simulink model "AFSK"  (R2024b)
settings: Solver=VariableStepAuto  StartTime=0  StopTime=phi_LOS.Time(end)  RelTol=1e-3
PreLoadFcn:
  | addpath('./inputs')
  | 
  | fc = 120e3;
  | delta_f = 1000; % Hz
  | f0 = fc-(delta_f/2);
  | f1 = fc+(delta_f/2);
  | 
  | Rb = 1200; % bit rate = 1,2 kbps
  | Tb = 1/Rb; % Bit period = Frame period
  | Nc = 4; % the number of samples between 0 and 2π of the carrier. There are 100 periods in each Ns samples.
  | Ns = fc*Tb*Nc; % = 400 The number of samples per Tb.
  | Tsamp = Tb/Ns; % Sample period
  | Rsamp = 1/Tsamp; % sampling rate
  | 
  | fd = delta_f/2; % Frequency deviation
  | h = 2*fd*Tb; % Indice de modulação (h=5/6)
  | 
  | impulse_response = get_matched_filter_impulse_response(Tsamp, Tb, Ns, h);
  | [all_phases, odd_phases, even_phases] = get_phases(h);
  | % `terminal_phases` is `all_phases` reshaped to be used
  | % in the Viterbi algorithm during the metric computation
  | terminal_phases = repmat(cat(3, odd_phases.', even_phases.'), [1, 2, 1]);
  | N_terminal_phases = length(all_phases);
  | % Viterbi delay
  | K = 25;
  | 
  | % uplink frequency
  | f_uplink = 149e6;
  | 
  | % get real satellite orbits from `scintpy`
  | scenarios = get_scenarios();
  | %% Programmatically changable settings
  | % NOTE: don't put these variables in InitFcn. Otherwise,
  | % programmatic simulations will not work. If you want
  | % to change these varuables manually, use the command
  | % window, instead.
  | scenario = scenarios(1);
  | is_Doppler_realistic = true;
InitFcn:
  | % get realistic ϕ_LOS (in rad) and tau_LOS (in sec) (both sampled in Tb)
  | [phi_LOS, tau_LOS]= get_LOS_effects(f_uplink, scenario, Tb);
  | % get initial estimates
  | initial_estimates = get_initial_estimates(phi_LOS.Data, Tb);
  | % tau in number of symbols (unitless, sampled  in Tb)
  | tau_LOS_symbols = tau_LOS/Tb;
  | % 𝜏 LOS in in number of samples (unitless, sampled in Tb)
  | tau_LOS_samples = tau_LOS_symbols*Ns;
  | 
  | % you can change it in the manual switch
  | EbN0 = str2double(get_param('AFSK/AWGN Channel', 'EbNo'));
  | 
  | %% Kalman filter configurations
  | 
  | if is_Doppler_realistic
  |     x_00 = initial_estimates;
  | 
  |     % The transmmitted bit is delayed by `(init_LOS_delay+1)*Tb`
  |     % seconds to be it is compared with the detected bits,
  |     % where `init_LOS_delay` is the floor of the maximum LOS
  |     % delay that happens during the simulation. The delay
  |     % estimation operates to estimate the (likely) fractional
  |     % part between `(init_LOS_delay+1)*Tb` and the real LOS delay
  |     % that is occuring. This difference is fed back so that the
  |     % receive is (ideally) always delayed in `(init_LOS_delay+1)*Tb`
  |     % seconds as well. When it happens, the timing delay
  |     % estimation is working in lock.
  |     init_LOS_delay = floor(max(tau_LOS_symbols.Data));
  | 
  |     fprintf("The satellite name run in Simulnk model is %s\n", scenario.sat_name);
  | else
  |     nu_synthetic = str2double(get_param('AFSK/nu', 'Value'));
  |     nu_dot_synthetic = str2double(get_param('AFSK/nu_dot', 'Value'));
  |     x_00 = [0 nu_synthetic nu_dot_synthetic];
  |     init_LOS_delay = 0;
  | 
  |     fprintf("Simulnk model is running for dummy scenario with Doppler shift and drift given by %d Hz and %d Hz/s,respectively\n",...
  |         nu_synthetic, nu_dot_synthetic);
  | end
  | 
  | % Taylor Series truncation order
  | M = 3;
  | sigma2_process = [zeros(1,M-1),1e-2];
  | [Px_0_0,x00_matrix,Fk,Qk,Hk,Rk] = get_kf_intial_cfg(EbN0, M, Tb, sigma2_process, x_00, init_LOS_delay);
undefined symbols (not defined in the file): all_phases, dspblkCoreblockFVToolHelper, Fk, gcbh, Hk, phi, Px_0_0, Qk, real_tau_LOS, Rk, x00_matrix
libraries: dspswit3 x8, dspstat3 x4, simulink x4, dspsigops x2, commchan3 x1, commrandsrc3 x1, dspfdesign x1, dspinverses x1, commsink2 x1
settings Model: SimulationMode=rapid-accelerator  Creator=Rubem Pacelli  LastModifiedBy=felix
settings SolverCC: AlgebraicLoopSolver=TrustRegion
settings DataIOCC: SaveFormat=Structure  SaveOutput=off  SignalLogging=off  DSMLogging=off  SaveTime=off  ReturnWorkspaceOutputs=off
settings DebuggingCC: UnconnectedInputMsg=warning  UnconnectedOutputMsg=warning  UnconnectedLineMsg=warning  ArithmeticOperatorsInVariantConditions=warning
settings ModelReferenceCC: EnableRefExpFcnMdlSchedulingChecks=on
settings SFSimCC: SimUseLocalCustomCode=off  CustomCodeUndefinedFunction=UseInterfaceOnly
settings RTWCC: RTWUseLocalCustomCode=off  GPUComputeCapability=3.5  DLArmComputeVersion=19.05

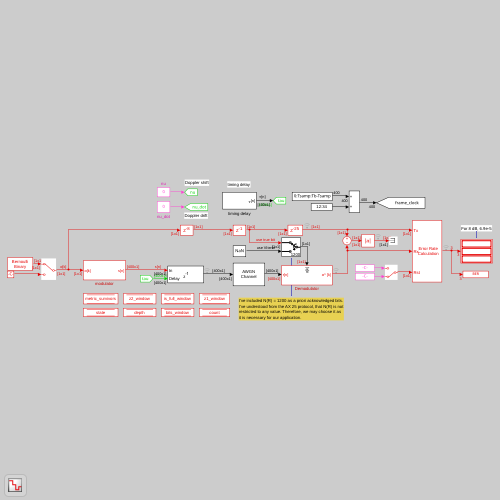
[thumbnail: Simulink's stored preview of the top-level diagram]
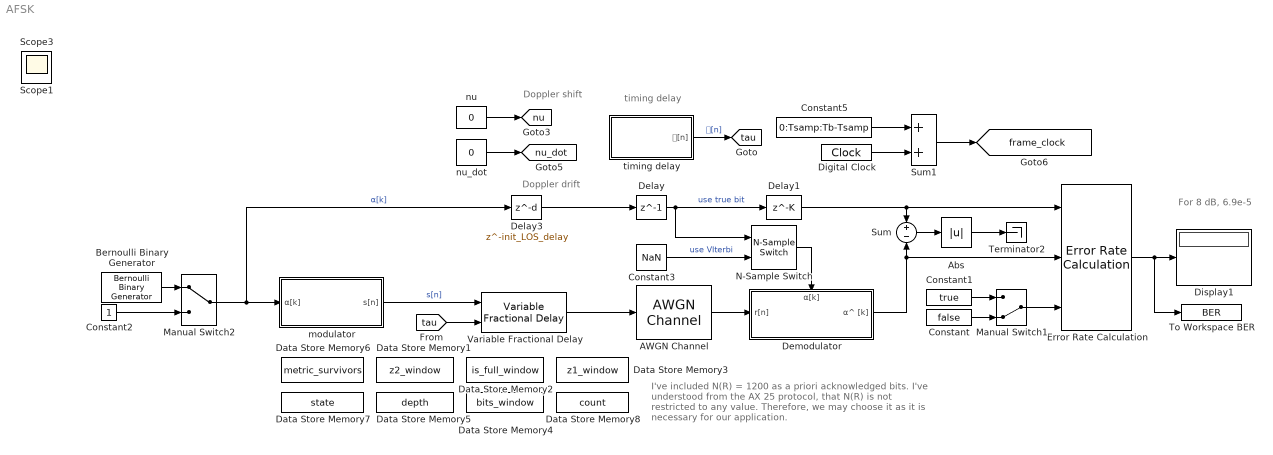
== system AFSK ==
  note: I've included N(R) = 1200 as a priori acknowledged bits.
      | I've understood from the AX 25 protocol, that N(R) is not
      | restricted to any value. Therefore, we may choose it as
      | it is necessary for our application.
  note: For 8 dB, 6.9e-5
  note: timing delay
  note: Doppler drift
  note: Doppler shift
  AWGN Channel : commchan3/AWGN Channel  LegacyMode=on  NoiseMethod="Signal to noise ratio  (SNR)"  noiseMode="Signal to noise ratio  (Eb/No)"  EbNo=12  EsNo=0  SNR=9  BitsPerSymbol=1  SignalPower=1  SamplesPerSymbol=1  SymbolPeriod=Tb  VarianceSource=Parameter  Variance=1  RandomStream=Global stream  Seed=10  SimulateUsing=Code generation
  Abs : Abs  SaturateOnIntegerOverflow=off
  Bernoulli Binary Generator : commrandsrc3/Bernoulli Binary Generator  ProbabilityOfZero=0.5  SeedSource=Parameter  Seed=10  SampleTime=Tb  SamplesPerFrame=1  OutputDataType=double  SimulateUsing=Interpreted execution
  Constant : Constant  Value=false
  Constant1 : Constant  Value=true
  Constant2 : Constant  SampleTime=Tb
  Constant3 : Constant  Value=NaN
  Constant5 : Constant  Value=0:Tsamp:Tb-Tsamp
  Data Store Memory1 : DataStoreMemory  DataStoreName=z2_window  ReadBeforeWriteMsg=warning  WriteAfterWriteMsg=warning  WriteAfterReadMsg=warning  InitialValue=NaN(N_terminal_phases/2, K)  ShowAdditionalParam=off  OutDataTypeStr=double  Dimensions=[N_terminal_phases/2 K]
      settings: SignalType=complex
  Data Store Memory2 : DataStoreMemory  DataStoreName=is_full_window  ReadBeforeWriteMsg=warning  WriteAfterWriteMsg=warning  WriteAfterReadMsg=warning  InitialValue=logical(0)  ShowAdditionalParam=off  OutDataTypeStr=boolean  Dimensions=1
  Data Store Memory3 : DataStoreMemory  DataStoreName=z1_window  ReadBeforeWriteMsg=warning  WriteAfterWriteMsg=warning  WriteAfterReadMsg=warning  InitialValue=NaN(N_terminal_phases/2, K)  ShowAdditionalParam=off  OutDataTypeStr=double  Dimensions=[N_terminal_phases/2 K]
      settings: SignalType=complex
  Data Store Memory4 : DataStoreMemory  DataStoreName=bits_window  ReadBeforeWriteMsg=warning  WriteAfterWriteMsg=warning  WriteAfterReadMsg=warning  InitialValue=5*ones(N_terminal_phases/2, K)  ShowAdditionalParam=off  OutDataTypeStr=double  Dimensions=[N_terminal_phases/2 K]
  Data Store Memory5 : DataStoreMemory  DataStoreName=depth  ReadBeforeWriteMsg=warning  WriteAfterWriteMsg=warning  WriteAfterReadMsg=warning  InitialValue=-init_LOS_delay  ShowAdditionalParam=off  OutDataTypeStr=double  Dimensions=1
  Data Store Memory6 : DataStoreMemory  DataStoreName=metric_survivors  ReadBeforeWriteMsg=warning  WriteAfterWriteMsg=warning  WriteAfterReadMsg=warning  InitialValue=zeros(1,N_terminal_phases/2)  ShowAdditionalParam=off  OutDataTypeStr=double  Dimensions=N_terminal_phases/2
  Data Store Memory7 : DataStoreMemory  DataStoreName=state  ReadBeforeWriteMsg=warning  WriteAfterWriteMsg=warning  WriteAfterReadMsg=warning  InitialValue=false  ShowAdditionalParam=off  OutDataTypeStr=boolean  Dimensions=1
  Data Store Memory8 : DataStoreMemory  DataStoreName=count  ReadBeforeWriteMsg=warning  WriteAfterWriteMsg=warning  WriteAfterReadMsg=warning  InitialValue=1  ShowAdditionalParam=off  OutDataTypeStr=double  Dimensions=1
  Delay : Delay  DelayLength=1  InitialCondition=NaN
  Delay1 : Delay  DelayLength=K  InitialCondition=NaN
  Delay3 : Delay  DelayLength=init_LOS_delay  InitialCondition=NaN
  Demodulator : Subsystem
      settings: PortSchema="{\"entries\":[{\"content\":{\"sides\":[{\"content\":{\"connectorIds\":[\"In1\"]},\"type\":\"ConnectorPlacement.EquallySpacedRectSide\",\"uuid\":\"ecba8ed6-bc33-46f0-af25-b274c72623b2\"},{\"content\":{\"connectorIds\":[\"Out1\"],\"side\":\"RIGHT\"},\"type\":\"ConnectorPlacement.EquallySpacedRectSide\",\"uuid\":\"d7f95e6f-fba9-4d7d-8ac9-e609210cafa8\"},{\"content\":{\"connectorIds\":[\"In2\"],\"side\":\"TOP\"},\"type\":\"ConnectorPlacement.EquallySpacedRectSide\",\"uuid\":\"b4a38cd2-b9d7-488f-8b29-7139030da35e\"}]},\"type\":\"ConnectorPlacement.EquallySpacedConnector\",\"uuid\":\"c7e86f76-54af-475b-ba8f-41016bad8b16\"}],\"packageUris\":[\"http://schema.mathworks.com/mf0/Connector/R2020b\"],\"version\":\"1.0\"}"
  Digital Clock : DigitalClock  SampleTime=Tb
  Display1 : Display
      settings: Format=short_e
  Error Rate Calculation : commsink2/Error Rate Calculation  N=0  st_delay=3.5e3  cp_mode=Entire frame  subframe=[]  PMode=Port  WsName=ErrorVec  RsMode2=on  stop=off  numErr=inf  maxBits=inf
  Manual Switch1 : ManualSwitch  CurrentSetting=0
  Manual Switch2 : ManualSwitch
  N-Sample Switch : dspswit3/N-Sample Switch  N=1200  reset=off  TriggerType=Rising edge  Ts=Tb
  Sum : Sum  Inputs=+-
  Sum1 : Sum
  Terminator2 : Terminator
  To Workspace BER : ToWorkspace  VariableName=BER  SampleTime=-1
      settings: MaxDataPoints=1
  Variable Fractional Delay : dspsigops/Variable Fractional Delay  mode=OBSOLETE  modeActive=Linear  L=4  FarrowL=4  R=10  alpha=1  dmax=ceil(max(tau_LOS_samples.Data))  InputProcessing=Columns as channels (frame based)  ic=0  noDFT=off  fallbackFIR=Clip to the minimum value necessary for centered kernel  fallbackFarrow=Clip to the minimum value necessary for centered kernel  roundingMode=Zero  overflowMode=off
  modulator : Subsystem
  nu : Constant  Value=0
  nu_dot : Constant  Value=0
  timing delay : Subsystem
  Scope1 : Scope
  Scope3 : Scope
  tag scope: frame_clock=global, nu=global, nu_dot=global, tau=global
  wires:
  Manual Switch2/1 -> Delay3/1, modulator/1(α[k])  "α[k]"
  AWGN Channel/1 -> Demodulator/1(r[n])
  Delay1/1 -> Error Rate Calculation/1, Sum/1
  Demodulator/1(α^ [k]) -> Error Rate Calculation/2, Sum/2
  Error Rate Calculation/1 -> Display1/1, To Workspace BER/1
  Variable Fractional Delay/1 -> AWGN Channel/1
  Sum/1 -> Abs/1
  Abs/1 -> Terminator2/1
  Manual Switch1/1 -> Error Rate Calculation/3
  Constant/1 -> Manual Switch1/2
  Constant1/1 -> Manual Switch1/1
  Bernoulli Binary Generator/1 -> Manual Switch2/1
  Delay/1 -> Delay1/1, N-Sample Switch/1  "use true bit"
  Constant2/1 -> Manual Switch2/2
  N-Sample Switch/1 -> Demodulator/2(α[k])
  Constant3/1 -> N-Sample Switch/2  "use VIterbi"
  Sum1/1 -> [frame_clock]
  nu/1 -> [nu]
  nu_dot/1 -> [nu_dot]
  Constant5/1 -> Sum1/1
  Digital Clock/1 -> Sum1/2
  Delay3/1 -> Delay/1
  [tau] -> Variable Fractional Delay/2
  modulator/1(s[n]) -> Variable Fractional Delay/1  "s[n]"
  timing delay/1(𝜏[n]) -> [tau]  "𝜏[n]"

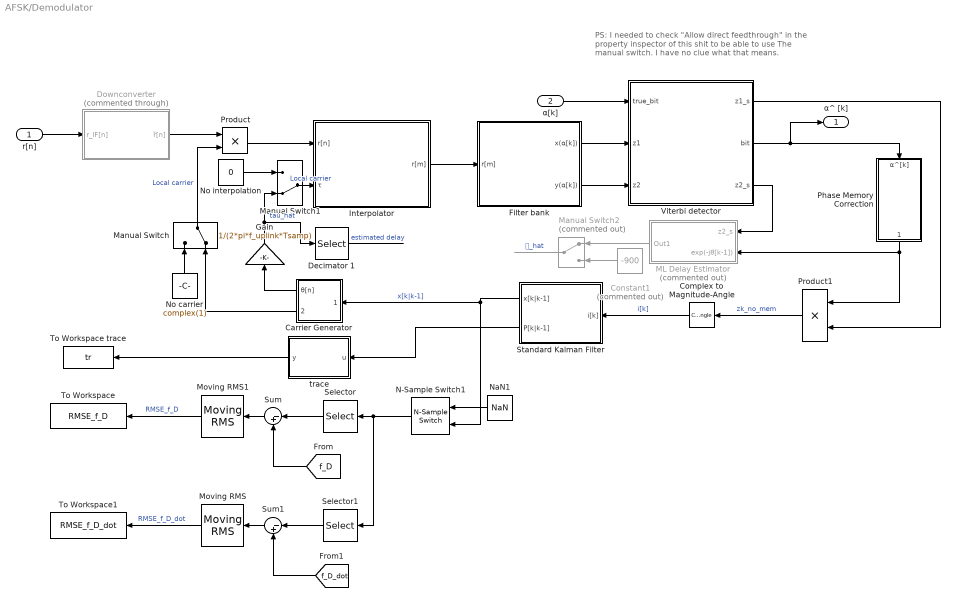
== system AFSK/Demodulator ==
  note: PS: I needed to check "Allow direct feedthrough"
      | in the property inspector of this shit to be able to use
      | The manual switch. I have no clue what that means.
  r[n] : Inport
  α[k] : Inport  Port=2
  Carrier Generator : Subsystem
  Complex to Magnitude-Angle : ComplexToMagnitudeAngle  Output=Angle
  Constant1 : Constant  Commented=on  Value=-900
  Decimator 1 : Selector  NumberOfDimensions=2  InputPortWidth=3  IndexOptions=Index vector (dialog),Select all  Indices=Ns,1  OutputSizes=1,1
  Downconverter : Subsystem  Commented=through
  Filter bank : Subsystem
  Gain : Gain  Gain=1/(2*pi*f_uplink*Tsamp)
  Interpolator : Subsystem
  ML Delay Estimator : Subsystem  Commented=on
  Manual Switch : ManualSwitch  CurrentSetting=0
  Manual Switch1 : ManualSwitch  CurrentSetting=0
  Manual Switch2 : ManualSwitch  Commented=on
  Moving RMS : dspstat3/Moving RMS  Method=Sliding window  ForgettingFactorPort=off  SpecifyWindowLength=on  WindowLength=3600  OverlapLength=3600-1  AllowArbitraryInputLength=off  ForgettingFactor=0.9  SimulateUsing=Interpreted execution
  Moving RMS1 : dspstat3/Moving RMS  Method=Sliding window  ForgettingFactorPort=off  SpecifyWindowLength=on  WindowLength=3600  OverlapLength=3600-1  AllowArbitraryInputLength=off  ForgettingFactor=0.9  SimulateUsing=Interpreted execution
  N-Sample Switch1 : dspswit3/N-Sample Switch  N=4  reset=off  TriggerType=Rising edge  Ts=Tb
  NaN1 : Constant  Value=NaN  OutDataTypeStr=Inherit: Inherit via back propagation
  No carrier : Constant  Value=complex(1)
  No interpolation : Constant  Value=0
  Phase Memory Correction : Subsystem
  Product : Product
  Product1 : Product
  Selector : Selector  InputPortWidth=3  IndexOptions=Index vector (dialog)  Indices=2  OutputSizes=1
  Selector1 : Selector  InputPortWidth=3  IndexOptions=Index vector (dialog)  Indices=3  OutputSizes=1
  Standard Kalman Filter : Subsystem
  Sum : Sum  Inputs=|-+
  Sum1 : Sum  Inputs=|-+
  To Workspace : ToWorkspace  VariableName=RMSE_f_D  SaveFormat=Timeseries  SampleTime=-1
  To Workspace trace : ToWorkspace  VariableName=tr  SaveFormat=Timeseries  SampleTime=-1
  To Workspace1 : ToWorkspace  VariableName=RMSE_f_D_dot  SaveFormat=Timeseries  SampleTime=-1
  Viterbi detector : MATLAB Function  TreatAsAtomicUnit=on
  trace : MATLAB Function  TreatAsAtomicUnit=on
  α^ [k] : Outport  VectorParamsAs1DForOutWhenUnconnected=off
  wires:
  Viterbi detector/2(bit) -> Phase Memory Correction/1(α^[k]), α^ [k]/1
  r[n]/1 -> Downconverter/1(r_IF[n])
  Interpolator/1(r[m]) -> Filter bank/1(r[m])
  Filter bank/2(y(α[k])) -> Viterbi detector/3(z2)
  Filter bank/1(x(α[k])) -> Viterbi detector/2(z1)
  Downconverter/1(r̃[n]) -> Product/1
  Product/1 -> Interpolator/1(r[n])
  Product1/1 -> Complex to Magnitude-Angle/1  "zk_no_mem"
  Viterbi detector/1(z1_s) -> Product1/2
  Complex to Magnitude-Angle/1 -> Standard Kalman Filter/1(i[k])  "i[k]"
  Standard Kalman Filter/1(x[k|k-1]) -> N-Sample Switch1/2, Carrier Generator/1(xkk1)  "x[k|k-1]"
  α[k]/1 -> Viterbi detector/1(true_bit)
  Constant1/1 -> Manual Switch2/2
  Manual Switch/1 -> Product/2  "Local carrier"
  Viterbi detector/3(z2_s) -> ML Delay Estimator/1(z2_s)
  ML Delay Estimator/1(Out1) -> Manual Switch2/1
  Phase Memory Correction/1(exp(-jθ[k-1])) -> Product1/1, ML Delay Estimator/2(exp(-jθ[k-1]))
  No carrier/1 -> Manual Switch/1
  Standard Kalman Filter/2(P[k|k-1]) -> trace/1(u)
  Carrier Generator/2(exp(-jθ[n])) -> Manual Switch/2
  Carrier Generator/1(θ[n]) -> Gain/1
  Manual Switch2/1 -> ?  "𝜏_hat"
  Gain/1 -> Manual Switch1/2, Decimator 1/1  "tau_hat"
  trace/1(y) -> To Workspace trace/1
  NaN1/1 -> N-Sample Switch1/1
  Selector/1 -> Sum/1
  [f_D] -> Sum/2
  [f_D_dot] -> Sum1/2
  Selector1/1 -> Sum1/1
  N-Sample Switch1/1 -> Selector1/1, Selector/1
  Sum1/1 -> Moving RMS/1
  Moving RMS/1 -> To Workspace1/1  "RMSE_f_D_dot"
  Moving RMS1/1 -> To Workspace/1  "RMSE_f_D"
  Sum/1 -> Moving RMS1/1
  Decimator 1/1 -> ?  "estimated delay"
  No interpolation/1 -> Manual Switch1/1
  Manual Switch1/1 -> Interpolator/2(τ)  "Local carrier"

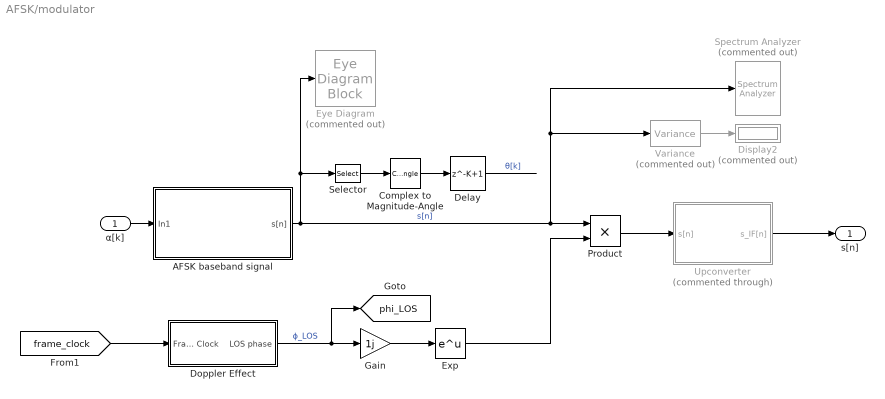
== system AFSK/modulator ==
  α[k] : Inport
  AFSK baseband signal : Subsystem
  Complex to Magnitude-Angle : ComplexToMagnitudeAngle  Output=Angle
  Delay : Delay  DelayLength=K+1  InitialCondition=NaN
  Display2 : Display  Commented=on
  Doppler Effect : Subsystem
  Exp : Math
  Eye Diagram : EyeDiagramBlock  Commented=on  WindowPosition=[1.000000,1.000000,1920.000000,1080.000000,]  ScopeFrameLocation=window  SamplesPerSymbol=Ns  SymbolsPerTrace=5  TracesToDisplay=100  Title=Phase trellis  YLimits=[-3.93,35.34]  PlotImaginaryAxes=off
      settings: OpenAtSimulationStart=off
  Gain : Gain  Gain=1j
  Product : Product
  Selector : Selector  InputPortWidth=Ns  IndexOptions=Index vector (dialog)  Indices=[Ns]  OutputSizes=1
  Spectrum Analyzer : SpectrumAnalyzer  Commented=on  WindowPosition=[1.000000,1.000000,1920.000000,1080.000000,]  ScopeFrameLocation=window  SpectrumType=Power density  Method=Welch  SampleRate=480000  PlotAsTwoSidedSpectrum=off  AxesScaling=Manual  FrequencySpan=Start and stop frequencies  StartFrequency=117e3  StopFrequency=123e3  AveragingMethod=Running  SpectralAverages=100  SpectrumUnits=dBm/Hz  Title=Spectrum of digital AFSK modulator  YLimits=[-70,22.62963183]  ExpandToolstrip=on  AllowFFTLengthLessThanSamplesPerUpdate=on
      settings: OpenAtSimulationStart=off
  Upconverter : Subsystem  Commented=through
  Variance : dspstat3/Variance  Commented=on  run=on  InputProcessing=Columns as channels (frame based)  reset_popup=None  directionMode=Each column  dimension=1  roiEnable=off  roiType=Rectangles  roiPortion=Entire ROI  roiOutput=Individual statistics for each ROI  roiFlag=off  roundingMode=Floor  overflowMode=off
  s[n] : Outport  VectorParamsAs1DForOutWhenUnconnected=off
  tag scope: phi_LOS=global
  wires:
  α[k]/1 -> AFSK baseband signal/1(In1)
  AFSK baseband signal/1(s[n]) -> Selector/1, Eye Diagram/1, Product/1, Variance/1, Spectrum Analyzer/1  "s[n]"
  Variance/1 -> Display2/1
  Selector/1 -> Complex to Magnitude-Angle/1
  Complex to Magnitude-Angle/1 -> Delay/1
  Delay/1 -> ?  "θ[k]"
  [frame_clock] -> Doppler Effect/1(Frame Clock)
  Doppler Effect/1(LOS phase) -> [phi_LOS], Gain/1  "ϕ_LOS"
  Product/1 -> Upconverter/1(s[n])
  Gain/1 -> Exp/1
  Exp/1 -> Product/2
  Upconverter/1(s_IF[n]) -> s[n]/1

== system AFSK/timing delay ==
  Constant : Constant  Value=is_Doppler_realistic
  Delay : Delay  DelayLength=1  InitialCondition=tau_LOS_symbols.Data(1)
  From Workspace : FromWorkspace  VariableName=tau_LOS_samples  SampleTime=-1  OutputAfterFinalValue=Holding final value
  Gain : Gain  Gain=-1
  Gain1 : Gain  Gain=1/(2*pi*f_uplink*Tsamp)
  Linear Interpolation : MATLAB Function  TreatAsAtomicUnit=on
  Switch : Switch  Criteria=u2 ~= 0  SaturateOnIntegerOverflow=off  InputSameDT=off
  𝜏[n] : Outport
  wires:
  Delay/1 -> Linear Interpolation/2(data_delayed)
  Linear Interpolation/1(y) -> Switch/1  "real 𝜏[n]"
  Gain/1 -> ?  "𝜏[k]"
  From Workspace/1 -> Delay/1, Linear Interpolation/1(data), Gain/1  "𝜏[k]"
  Constant/1 -> Switch/2
  Gain1/1 -> Switch/3  "synthetic 𝜏[n]"
  [phi_LOS] -> Gain1/1
  Switch/1 -> 𝜏[n]/1  "𝜏[n]"

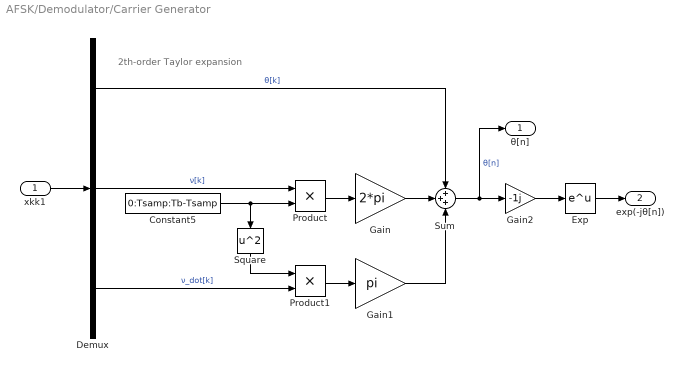
== system AFSK/Demodulator/Carrier Generator ==
  note: 2th-order Taylor expansion
  xkk1 : Inport
  Constant5 : Constant  Value=0:Tsamp:Tb-Tsamp
  Demux : Demux  Outputs=3
  Exp : Math
  Gain : Gain  Gain=2*pi
  Gain1 : Gain  Gain=pi
  Gain2 : Gain  Gain=-1j
  Product : Product
  Product1 : Product
  Square : Math  Operator=square
  Sum : Sum  Inputs=+++
  θ[n] : Outport
  exp(-jθ[n]) : Outport  Port=2
  wires:
  Exp/1 -> exp(-jθ[n])/1
  Gain2/1 -> Exp/1
  xkk1/1 -> Demux/1
  Demux/2 -> Product/1  "ν[k]"
  Sum/1 -> θ[n]/1, Gain2/1  "θ[n]"
  Demux/1 -> Sum/1  "θ[k]"
  Constant5/1 -> Square/1, Product/2
  Product/1 -> Gain/1
  Gain/1 -> Sum/2
  Product1/1 -> Gain1/1
  Demux/3 -> Product1/2  "ν_dot[k]"
  Square/1 -> Product1/1
  Gain1/1 -> Sum/3

== system AFSK/Demodulator/Downconverter ==
  r_IF[n] : Inport
  Digital Filter Design1 : dspfdesign/Digital Filter Design  mwdsp_browser_bugfix_var=off
  Gain : Gain  Gain=sqrt(2)
  Local oscilator : Subsystem
  Product : Product
  r̃[n] : Outport
  wires:
  r_IF[n]/1 -> Product/2
  Local oscilator/1(Out1) -> Product/1
  Product/1 -> Digital Filter Design1/1
  Digital Filter Design1/1 -> Gain/1
  Gain/1 -> r̃[n]/1

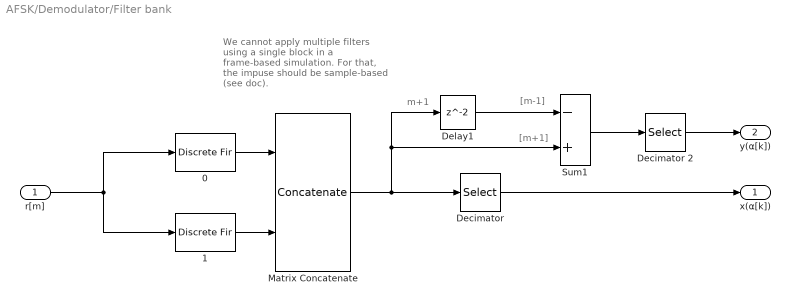
== system AFSK/Demodulator/Filter bank ==
  note: We cannot apply multiple filters using a single block in a
      | frame-based simulation. For that,
      | the impuse should be sample-based (see doc).
  note: [m-1]
  note: [m+1]
  note: m+1
  r[m] : Inport
  0 : DiscreteFir  LoadFcn=dspblkCoreblockFVToolHelper(gcbh,'load');  Coefficients=flip(impulse_response(:,1)')  InputProcessing=Columns as channels (frame based)
      settings: CopyFcn=dspblkCoreblockFVToolHelper(gcbh,'copy');  DeleteFcn=dspblkCoreblockFVToolHelper(gcbh,'close');  ModelCloseFcn=dspblkCoreblockFVToolHelper(gcbh,'close');  PreSaveFcn=dspblkCoreblockFVToolHelper(gcbh,'presave');  PostSaveFcn=dspblkCoreblockFVToolHelper(gcbh,'postsave');  CloseFcn=dspblkCoreblockFVToolHelper(gcbh,'close');
  1 : DiscreteFir  LoadFcn=dspblkCoreblockFVToolHelper(gcbh,'load');  Coefficients=flip(impulse_response(:,2)')  InputProcessing=Columns as channels (frame based)
      settings: CopyFcn=dspblkCoreblockFVToolHelper(gcbh,'copy');  DeleteFcn=dspblkCoreblockFVToolHelper(gcbh,'close');  ModelCloseFcn=dspblkCoreblockFVToolHelper(gcbh,'close');  PreSaveFcn=dspblkCoreblockFVToolHelper(gcbh,'presave');  PostSaveFcn=dspblkCoreblockFVToolHelper(gcbh,'postsave');  CloseFcn=dspblkCoreblockFVToolHelper(gcbh,'close');
  Decimator : Selector  NumberOfDimensions=2  InputPortWidth=3  IndexOptions=Index vector (dialog),Select all  Indices=Ns,Ns  OutputSizes=1,1
  Decimator 2 : Selector  NumberOfDimensions=2  InputPortWidth=3  IndexOptions=Index vector (dialog),Select all  Indices=Ns,1  OutputSizes=1,1
  Delay1 : Delay  InputProcessing=Columns as channels (frame based)
  Matrix Concatenate : Concatenate  Mode=Multidimensional array  ConcatenateDimension=2
  Sum1 : Sum  Inputs=-+
  x(α[k]) : Outport
  y(α[k]) : Outport  Port=2
  wires:
  r[m]/1 -> 1/1, 0/1
  1/1 -> Matrix Concatenate/2
  0/1 -> Matrix Concatenate/1
  Sum1/1 -> Decimator 2/1
  Delay1/1 -> Sum1/1
  Decimator 2/1 -> y(α[k])/1
  Decimator/1 -> x(α[k])/1
  Matrix Concatenate/1 -> Delay1/1, Sum1/2, Decimator/1

== system AFSK/Demodulator/Interpolator ==
  note: Make this dynamic
  r[n] : Inport
  τ : Inport  Port=2
  Bias1 : Bias  Bias=(init_LOS_delay+1)*Ns  SaturateOnIntegerOverflow=off
  Delay : Delay  Commented=on  DelayLengthSource=Input port  DelayLength=Ns-9  DelayLengthUpperLimit=Ns-9  InputProcessing=Columns as channels (frame based)
      settings: InputPortMap=u0,p1
  Selector : Selector  Commented=on  NumberOfDimensions=2  InputPortWidth=3  IndexOptions=Select all,Index vector (dialog)  Indices=[1 3],1  OutputSizes=1,1
  Variable Fractional Delay : dspsigops/Variable Fractional Delay  mode=OBSOLETE  modeActive=Farrow  L=4  FarrowL=10  R=10  alpha=1  dmax=ceil(max(tau_LOS_samples.Data))  InputProcessing=Columns as channels (frame based)  ic=0  noDFT=off  fallbackFIR=Clip to the minimum value necessary for centered kernel  fallbackFarrow=Clip to the minimum value necessary for centered kernel  roundingMode=Zero  overflowMode=off
  r[m] : Outport
  wires:
  τ/1 -> Bias1/1
  Selector/1 -> ?
  Bias1/1 -> Variable Fractional Delay/2
  r[n]/1 -> Selector/1, Variable Fractional Delay/1
  Variable Fractional Delay/1 -> r[m]/1

== system AFSK/Demodulator/ML Delay Estimator ==
  z2_s : Inport
  exp(-jθ[k-1]) : Inport  Port=2
  Complex to Real-Imag : ComplexToRealImag  Output=Real
  Delay : Delay  DelayLength=1
  Delay1 : Delay  DelayLength=1
  Delay2 : Delay  DelayLength=1  InitialCondition=-real_tau_LOS.Data(1)
  Gain1 : Gain  Gain=1e-1
  Product2 : Product
  Sum : Sum  Inputs=|-+
  Out1 : Outport
  wires:
  z2_s/1 -> Delay/1
  Delay1/1 -> Product2/2
  Delay/1 -> Product2/1
  exp(-jθ[k-1])/1 -> Delay1/1
  Delay2/1 -> Sum/2
  Sum/1 -> Out1/1, Delay2/1
  Product2/1 -> Complex to Real-Imag/1
  Gain1/1 -> Sum/1
  Complex to Real-Imag/1 -> Gain1/1

== system AFSK/Demodulator/Phase Memory Correction ==
  note: θ[k] contains the phase memory unti the kth
      | symbol. However, for z[k], we need to remove
      | the memory until the k-1th symbol.
  α^[k] : Inport
  Delay : Delay  DelayLength=1
  Exp : Math
  Gain : Gain  Gain=-1j
  Terminal phase lookup table : Subsystem
  exp(-jθ[k-1]) : Outport
  wires:
  Delay/1 -> Gain/1
  Gain/1 -> Exp/1
  Terminal phase lookup table/1(θ^[k]) -> Delay/1  "θ^[k]"
  Exp/1 -> exp(-jθ[k-1])/1
  α^[k]/1 -> Terminal phase lookup table/1(α^ [k])

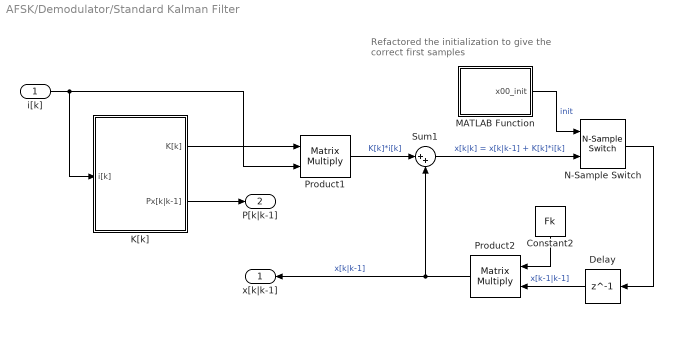
== system AFSK/Demodulator/Standard Kalman Filter ==
  note: Refactored the initialization
      | to give the correct first samples
  i[k] : Inport
  Constant2 : Constant  Value=Fk  VectorParams1D=off  SampleTime=Tb
  Delay : Delay  DelayLength=1  InitialCondition=0
  K[k] : Subsystem
  MATLAB Function : MATLAB Function  TreatAsAtomicUnit=on
  N-Sample Switch : dspswit3/N-Sample Switch  N=25 + init_LOS_delay + 1  reset=off  TriggerType=Rising edge  Ts=Tb
  Product1 : Product  Multiplication=Matrix(*)
  Product2 : Product  Multiplication=Matrix(*)
  Sum1 : Sum  Inputs=|++
  x[k|k-1] : Outport  VectorParamsAs1DForOutWhenUnconnected=off
  P[k|k-1] : Outport  Port=2
  wires:
  i[k]/1 -> K[k]/1(i[k]), Product1/2
  Constant2/1 -> Product2/1
  Product1/1 -> Sum1/1  "K[k]*i[k]"
  Product2/1 -> x[k|k-1]/1, Sum1/2  "x[k|k-1]"
  Delay/1 -> Product2/2  "x[k-1|k-1]"
  Sum1/1 -> N-Sample Switch/2  "x[k|k] = x[k|k-1] + K[k]*i[k]"
  N-Sample Switch/1 -> Delay/1
  K[k]/1(K[k]) -> Product1/1
  K[k]/2(Px[k|k-1]) -> P[k|k-1]/1
  MATLAB Function/1(x00_init) -> N-Sample Switch/1  "init"

== system AFSK/modulator/AFSK baseband signal ==
  In1 : Inport
  Exp : Math
  Gain1 : Gain  Gain=1j*2*pi*h
  Integrator : Subsystem
  mapping bit : Subsystem
  s[n] : Outport
  wires:
  In1/1 -> mapping bit/1(In)
  mapping bit/1(Out) -> Integrator/1(I[n])  "I[n]"
  Integrator/1(Out1) -> Gain1/1
  Gain1/1 -> Exp/1  "Φ[n]"
  Exp/1 -> s[n]/1

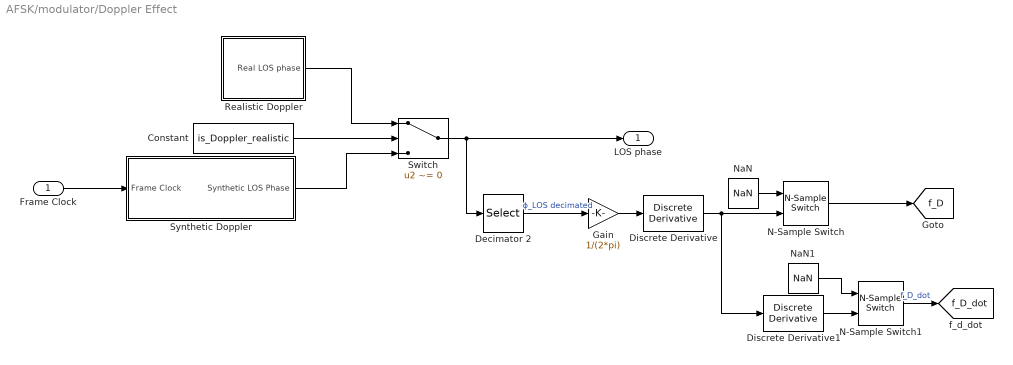
== system AFSK/modulator/Doppler Effect ==
  Frame Clock : Inport
  Constant : Constant  Value=is_Doppler_realistic
  Decimator 2 : Selector  NumberOfDimensions=2  InputPortWidth=3  IndexOptions=Index vector (dialog),Select all  Indices=Ns,1  OutputSizes=1,1
  Discrete Derivative : simulink/Discrete/Discrete Derivative  gainval=1.0  ICPrevScaledInput=0.0  OutMin=[]  OutMax=[]  OutDataType=fixdt(1, 16)  OutScaling=2^-10  DoSatur=off
  Discrete Derivative1 : simulink/Discrete/Discrete Derivative  gainval=1.0  ICPrevScaledInput=0.0  OutMin=[]  OutMax=[]  OutDataType=fixdt(1, 16)  OutScaling=2^-10  DoSatur=off
  Gain : Gain  Gain=1/(2*pi)
  N-Sample Switch : dspswit3/N-Sample Switch  N=4  reset=off  TriggerType=Rising edge  Ts=Tb
  N-Sample Switch1 : dspswit3/N-Sample Switch  N=4  reset=off  TriggerType=Rising edge  Ts=Tb
  NaN : Constant  Value=NaN  OutDataTypeStr=Inherit: Inherit via back propagation
  NaN1 : Constant  Value=NaN  OutDataTypeStr=Inherit: Inherit via back propagation
  Realistic Doppler : Subsystem
  Switch : Switch  Criteria=u2 ~= 0  SaturateOnIntegerOverflow=off  InputSameDT=off
  Synthetic Doppler : Subsystem
  LOS phase : Outport
  tag scope: f_D=global, f_D_dot=global
  wires:
  Frame Clock/1 -> Synthetic Doppler/1(Frame Clock)
  Constant/1 -> Switch/2
  Realistic Doppler/1(Real LOS phase) -> Switch/1
  Synthetic Doppler/1(Synthetic LOS Phase) -> Switch/3
  Switch/1 -> LOS phase/1, Decimator 2/1
  Decimator 2/1 -> Gain/1  "ϕ_LOS decimated"
  Discrete Derivative/1 -> N-Sample Switch/2, Discrete Derivative1/1
  NaN/1 -> N-Sample Switch/1
  NaN1/1 -> N-Sample Switch1/1
  Discrete Derivative1/1 -> N-Sample Switch1/2
  Gain/1 -> Discrete Derivative/1
  N-Sample Switch/1 -> [f_D]
  N-Sample Switch1/1 -> [f_D_dot]  "f_D_dot"

== system AFSK/modulator/Upconverter ==
  s[n] : Inport
  Carrier with Doppler : Subsystem
  Complex to Real-Imag : ComplexToRealImag  Output=Real
  Gain : Gain  Gain=sqrt(2)
  Product : Product
  s_IF[n] : Outport  VectorParamsAs1DForOutWhenUnconnected=off
  wires:
  Product/1 -> Complex to Real-Imag/1
  Carrier with Doppler/1(Out1) -> Product/1
  Complex to Real-Imag/1 -> Gain/1
  s[n]/1 -> Product/2
  Gain/1 -> s_IF[n]/1

== system AFSK/Demodulator/Downconverter/Local oscilator ==
  Constant : Constant  Value=fc
  Exp : Math
  Gain : Gain  Gain=-1j*2*pi
  Product2 : Product
  Out1 : Outport
  wires:
  Gain/1 -> Product2/2
  Constant/1 -> Gain/1
  Exp/1 -> Out1/1
  [frame_clock] -> Product2/1
  Product2/1 -> Exp/1

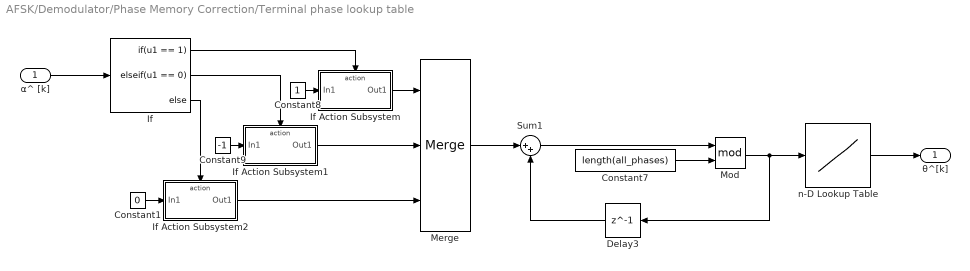
== system AFSK/Demodulator/Phase Memory Correction/Terminal phase lookup table ==
  α^ [k] : Inport
  Constant1 : Constant  Value=0
  Constant7 : Constant  Value=length(all_phases)
  Constant8 : Constant
  Constant9 : Constant  Value=-1
  Delay3 : Delay  DelayLength=1
  If : If  IfExpression=u1 == 1  ElseIfExpressions=u1 == 0
  If Action Subsystem : Subsystem  TreatAsAtomicUnit=on
  If Action Subsystem1 : Subsystem  TreatAsAtomicUnit=on
  If Action Subsystem2 : Subsystem  TreatAsAtomicUnit=on
  Merge : Merge  Inputs=3
  Mod : Math  Operator=mod
  Sum1 : Sum  Inputs=|++
  n-D Lookup Table : Lookup_n-D  NumberOfTableDimensions=1  LookupTableObject=''  BreakpointsForDimension1=0:length(all_phases)-1  BreakpointsForDimension2=[1:2]  BreakpointsForDimension3=[5, 7]  BreakpointsForDimension1FirstPoint=10  BreakpointsForDimension2FirstPoint=10  BreakpointsForDimension1Spacing=12  BreakpointsForDimension2Spacing=12  IndexSearchMethod=Evenly spaced points  Table=all_phases  InterpMethod=Flat  DiagnosticForOutOfRangeInput=Error  InternalRulePriority=Speed  RndMeth=Simplest
  θ^[k] : Outport
  wires:
  Sum1/1 -> Mod/1
  Constant9/1 -> If Action Subsystem1/1(In1)
  Constant8/1 -> If Action Subsystem/1(In1)
  Mod/1 -> n-D Lookup Table/1, Delay3/1
  n-D Lookup Table/1 -> θ^[k]/1
  Delay3/1 -> Sum1/2
  Constant7/1 -> Mod/2
  α^ [k]/1 -> If/1
  If/1 -> If Action Subsystem/Action
  If/2 -> If Action Subsystem1/Action
  If/3 -> If Action Subsystem2/Action
  Constant1/1 -> If Action Subsystem2/1(In1)
  If Action Subsystem2/1(Out1) -> Merge/3
  If Action Subsystem1/1(Out1) -> Merge/2
  If Action Subsystem/1(Out1) -> Merge/1
  Merge/1 -> Sum1/1

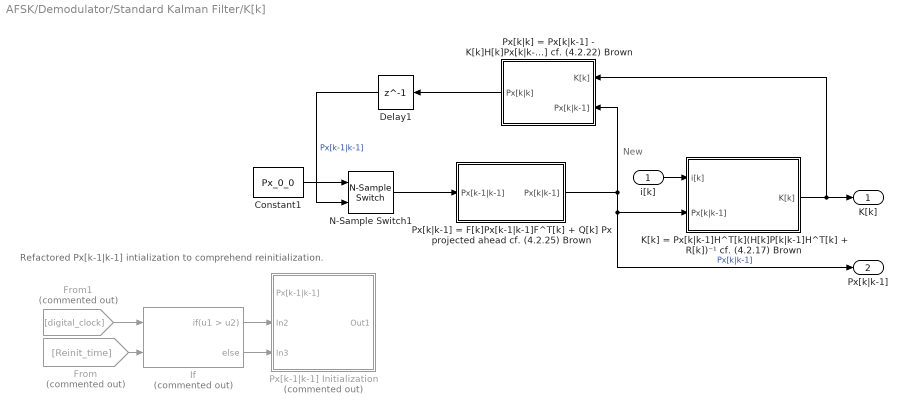
== system AFSK/Demodulator/Standard Kalman Filter/K[k] ==
  note: New
  note: Refactored Px[k-1|k-1] intialization
      | to comprehend reinitialization.
  i[k] : Inport
  Constant1 : Constant  Value=Px_0_0  VectorParams1D=off  SampleTime=Tb
  Delay1 : Delay  DelayLength=1  InitialCondition=0
  From : From  Commented=on  GotoTag=Reinit_time  TagVisibility=global
  From1 : From  Commented=on  GotoTag=digital_clock  TagVisibility=global
  If : If  Commented=on  NumInputs=2  IfExpression=u1 > u2
  K[k] = Px[k|k-1]H^T[k](H[k]P[k|k-1]H^T[k] + R[k])⁻¹ cf. (4.2.17) Brown : Subsystem
  N-Sample Switch1 : dspswit3/N-Sample Switch  N=26  reset=off  TriggerType=Rising edge  Ts=Tb
  Px[k-1|k-1] Initialization : Subsystem  Commented=on
  Px[k|k-1] = F[k]Px[k-1|k-1]F^T[k] + Q[k] Px projected ahead cf. (4.2.25) Brown : Subsystem
  Px[k|k] = Px[k|k-1] - K[k]H[k]Px[k|k-1] cf. (4.2.22) Brown : Subsystem
  K[k] : Outport  VectorParamsAs1DForOutWhenUnconnected=off
  Px[k|k-1] : Outport  Port=2
  wires:
  K[k] = Px[k|k-1]H^T[k](H[k]P[k|k-1]H^T[k] + R[k])⁻¹ cf. (4.2.17) Brown/1(K[k]) -> K[k]/1, Px[k|k] = Px[k|k-1] - K[k]H[k]Px[k|k-1] cf. (4.2.22) Brown/1(K[k])
  Px[k|k-1] = F[k]Px[k-1|k-1]F^T[k] + Q[k] Px projected ahead cf. (4.2.25) Brown/1(Px[k|k-1]) -> Px[k|k-1]/1, K[k] = Px[k|k-1]H^T[k](H[k]P[k|k-1]H^T[k] + R[k])⁻¹ cf. (4.2.17) Brown/2(Px[k|k-1]), Px[k|k] = Px[k|k-1] - K[k]H[k]Px[k|k-1] cf. (4.2.22) Brown/2(Px[k|k-1])  "Px[k|k-1]"
  N-Sample Switch1/1 -> Px[k|k-1] = F[k]Px[k-1|k-1]F^T[k] + Q[k] Px projected ahead cf. (4.2.25) Brown/1(Px[k-1|k-1])
  Px[k|k] = Px[k|k-1] - K[k]H[k]Px[k|k-1] cf. (4.2.22) Brown/1(Px[k|k]) -> Delay1/1
  i[k]/1 -> K[k] = Px[k|k-1]H^T[k](H[k]P[k|k-1]H^T[k] + R[k])⁻¹ cf. (4.2.17) Brown/1(i[k])
  If/1 -> Px[k-1|k-1] Initialization/2(In2)
  From1/1 -> If/1
  From/1 -> If/2
  If/2 -> Px[k-1|k-1] Initialization/3(In3)
  Constant1/1 -> N-Sample Switch1/1
  Delay1/1 -> N-Sample Switch1/2  "Px[k-1|k-1]"

== system AFSK/modulator/AFSK baseband signal/Integrator ==
  I[n] : Inport
  Constant : Constant  Value=linspace(Tsamp / (2*Tb),0.5,Ns)  SampleTime=Tb
  Constant1 : Constant  Value=-linspace(Tsamp / (2*Tb),0.5,Ns)  SampleTime=Tb
  Constant2 : Constant  Value=5/h  SampleTime=Tb
  Delay : Delay  DelayLength=1
  Selector : Selector  InputPortWidth=Ns  IndexOptions=Index vector (dialog)  Indices=[Ns]  OutputSizes=1
  Sum1 : Sum  Inputs=|++
  Switch : Switch  Criteria=u2 > Threshold  SaturateOnIntegerOverflow=off  InputSameDT=off
  fase entre -π e π : Math  Operator=mod  SignedPower=on
  Out1 : Outport  VectorParamsAs1DForOutWhenUnconnected=off
  wires:
  I[n]/1 -> Switch/2
  Selector/1 -> Delay/1
  Constant1/1 -> Switch/3
  Constant2/1 -> fase entre -π e π/2
  Constant/1 -> Switch/1
  fase entre -π e π/1 -> Out1/1, Selector/1
  Delay/1 -> Sum1/2
  Sum1/1 -> fase entre -π e π/1
  Switch/1 -> Sum1/1

== system AFSK/modulator/AFSK baseband signal/mapping bit ==
  In : Inport
  Constant : Constant  SampleTime=Tb
  Constant1 : Constant  Value=-1  SampleTime=Tb
  Switch : Switch  Criteria=u2 > Threshold  SaturateOnIntegerOverflow=off  InputSameDT=off
  Out : Outport  VectorParamsAs1DForOutWhenUnconnected=off
  wires:
  Constant/1 -> Switch/1
  Constant1/1 -> Switch/3
  In/1 -> Switch/2
  Switch/1 -> Out/1

== system AFSK/modulator/Doppler Effect/Realistic Doppler ==
  Delay : Delay  DelayLength=1  InitialCondition=initial_estimates(1)
  From Workspace : FromWorkspace  VariableName=phi_LOS  SampleTime=Tb
  Linear Interpolation : MATLAB Function  TreatAsAtomicUnit=on
  Real LOS phase : Outport
  wires:
  Linear Interpolation/1(y) -> Real LOS phase/1  "Real LOS phase"
  Delay/1 -> Linear Interpolation/2(data_delayed)
  From Workspace/1 -> Delay/1, Linear Interpolation/1(data)  "real LOS phase"

== system AFSK/modulator/Doppler Effect/Synthetic Doppler ==
  note: θ[n] ~= θ[0] + 2πν[n]nTs + 2πν[n](nTs)²/2
  note: 2th-order Taylor expansion
  Frame Clock : Inport
  Gain2 : Gain  Gain=2*pi
  Gain3 : Gain  Gain=pi
  Product1 : Product
  Product2 : Product
  Square : Math  Operator=square
  Sum2 : Sum  Inputs=++|
  Synthetic LOS Phase : Outport
  wires:
  [nu] -> Gain2/1
  Gain2/1 -> Product2/2
  Frame Clock/1 -> Square/1, Product2/1
  Product1/1 -> Sum2/1
  [nu_dot] -> Gain3/1
  Square/1 -> Product1/2
  Product2/1 -> Sum2/2
  Gain3/1 -> Product1/1
  Sum2/1 -> Synthetic LOS Phase/1  "LOS Phase"

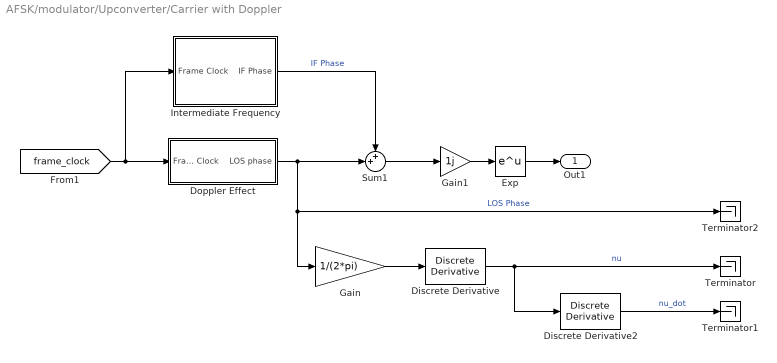
== system AFSK/modulator/Upconverter/Carrier with Doppler ==
  Discrete Derivative : simulink/Discrete/Discrete Derivative  gainval=Ns  ICPrevScaledInput=0  InputProcessing=Columns as channels (frame based)  OutMin=[]  OutMax=[]  OutDataType=fixdt(1, 16)  OutScaling=2^-10  DoSatur=off
  Discrete Derivative2 : simulink/Discrete/Discrete Derivative  gainval=Ns  ICPrevScaledInput=0  InputProcessing=Columns as channels (frame based)  OutMin=[]  OutMax=[]  OutDataType=fixdt(1, 16)  OutScaling=2^-10  DoSatur=off
  Doppler Effect : Subsystem
  Exp : Math
  Gain : Gain  Gain=1/(2*pi)
  Gain1 : Gain  Gain=1j
  Intermediate Frequency : Subsystem
  Sum1 : Sum  Inputs=++|
  Terminator : Terminator
  Terminator1 : Terminator
  Terminator2 : Terminator
  Out1 : Outport
  wires:
  Exp/1 -> Out1/1
  Gain1/1 -> Exp/1
  Sum1/1 -> Gain1/1
  [frame_clock] -> Doppler Effect/1(Frame Clock), Intermediate Frequency/1(Frame Clock)
  Intermediate Frequency/1(IF Phase) -> Sum1/1  "IF Phase"
  Gain/1 -> Discrete Derivative/1
  Discrete Derivative/1 -> Discrete Derivative2/1, Terminator/1  "nu"
  Discrete Derivative2/1 -> Terminator1/1  "nu_dot"
  Doppler Effect/1(LOS phase) -> Terminator2/1, Gain/1, Sum1/2  "LOS Phase"

== system AFSK/Demodulator/Phase Memory Correction/Terminal phase lookup table/If Action Subsystem ==
  In1 : Inport
  Action Port : ActionPort  ActionPortLabel=if(u1 == 1)
  Out1 : Outport
  wires:
  In1/1 -> Out1/1

== system AFSK/Demodulator/Phase Memory Correction/Terminal phase lookup table/If Action Subsystem1 ==
  In1 : Inport
  Action Port : ActionPort  ActionPortLabel=elseif(u1 == 0)
  Out1 : Outport
  wires:
  In1/1 -> Out1/1

== system AFSK/Demodulator/Phase Memory Correction/Terminal phase lookup table/If Action Subsystem2 ==
  In1 : Inport
  Action Port : ActionPort  ActionPortLabel=else
  Out1 : Outport
  wires:
  In1/1 -> Out1/1

== system AFSK/Demodulator/Standard Kalman Filter/K[k]/K[k] = Px[k|k-1]H^T[k](H[k]P[k|k-1]H^T[k] + R[k])⁻¹ cf. (4.2.17) Brown ==
  note: New
  i[k] : Inport
  Px[k|k-1] : Inport  Port=2
  " Pz[k|k-1] = H[k] Px[k|k-1] H^T[k] + R[k]" : Subsystem
  " LU Inverse" : dspinverses/ LU Inverse
  Constant7 : Constant  Value=Hk  VectorParams1D=off  SampleTime=Tb
  Product11 : Product  Inputs=3  Multiplication=Matrix(*)
  Transpose : Math  Operator=transpose
  K[k] : Outport  VectorParamsAs1DForOutWhenUnconnected=off
  wires:
  " LU Inverse"/1 -> Product11/3  "Pz^(-1)[k|k-1]"
  " Pz[k|k-1] = H[k] Px[k|k-1] H^T[k] + R[k]"/1(Pz[k|k-1]) -> " LU Inverse"/1
  Product11/1 -> K[k]/1
  Px[k|k-1]/1 -> " Pz[k|k-1] = H[k] Px[k|k-1] H^T[k] + R[k]"/1(Px[k|k-1]), Product11/1  "Px[k|k-1]"
  Constant7/1 -> Transpose/1
  Transpose/1 -> Product11/2
  i[k]/1 -> " Pz[k|k-1] = H[k] Px[k|k-1] H^T[k] + R[k]"/2(i[k])

== system AFSK/Demodulator/Standard Kalman Filter/K[k]/Px[k-1|k-1] Initialization ==
  Px[k-1|k-1] : Inport
  In2 : Inport  Port=2
  In3 : Inport  Port=3
  If Action Subsystem : Subsystem  TreatAsAtomicUnit=on
  If Action Subsystem1 : Subsystem  TreatAsAtomicUnit=on
  Merge : Merge
  Out1 : Outport
  wires:
  Px[k-1|k-1]/1 -> If Action Subsystem/1(In1), If Action Subsystem1/1(In1)
  In2/1 -> If Action Subsystem1/Action
  If Action Subsystem/1(Out1) -> Merge/2
  If Action Subsystem1/1(Out1) -> Merge/1
  Merge/1 -> Out1/1
  In3/1 -> If Action Subsystem/Action

== system AFSK/Demodulator/Standard Kalman Filter/K[k]/Px[k|k-1] = F[k]Px[k-1|k-1]F^T[k] + Q[k] Px projected ahead cf. (4.2.25) Brown ==
  Px[k-1|k-1] : Inport
  Constant : Constant  Value=Qk
  Constant4 : Constant  Value=Fk  VectorParams1D=off  SampleTime=Tb
  Product5 : Product  Inputs=3  Multiplication=Matrix(*)
  Sum2 : Sum  Inputs=|++
  Transpose : Math  Operator=transpose  SignedPower=on
  Px[k|k-1] : Outport  VectorParamsAs1DForOutWhenUnconnected=off
  wires:
  Product5/1 -> Sum2/1
  Constant4/1 -> Transpose/1, Product5/1
  Sum2/1 -> Px[k|k-1]/1  "Px[k|k-1]"
  Transpose/1 -> Product5/3
  Px[k-1|k-1]/1 -> Product5/2
  Constant/1 -> Sum2/2

== system AFSK/Demodulator/Standard Kalman Filter/K[k]/Px[k|k] = Px[k|k-1] - K[k]H[k]Px[k|k-1] cf. (4.2.22) Brown ==
  K[k] : Inport
  Px[k|k-1] : Inport  Port=2
  Constant7 : Constant  Value=Hk  VectorParams1D=off  SampleTime=Tb
  Product7 : Product  Inputs=3  Multiplication=Matrix(*)
  Sum4 : Sum  Inputs=|-+
  Px[k|k] : Outport  VectorParamsAs1DForOutWhenUnconnected=off
  wires:
  Sum4/1 -> Px[k|k]/1  "Px[k|k]"
  Product7/1 -> Sum4/1
  K[k]/1 -> Product7/1
  Px[k|k-1]/1 -> Product7/3, Sum4/2
  Constant7/1 -> Product7/2

== system AFSK/modulator/Upconverter/Carrier with Doppler/Doppler Effect ==
  Frame Clock : Inport
  Constant : Constant  Value=is_Doppler_realistic
  Realistic Doppler : Subsystem
  Switch : Switch  Criteria=u2 ~= 0  SaturateOnIntegerOverflow=off  InputSameDT=off
  Synthetic Doppler : Subsystem
  LOS phase : Outport
  wires:
  Frame Clock/1 -> Synthetic Doppler/1(Frame Clock)
  Constant/1 -> Switch/2
  Realistic Doppler/1(Real LOS phase) -> Switch/1
  Synthetic Doppler/1(Synthetic LOS Phase) -> Switch/3
  Switch/1 -> LOS phase/1

== system AFSK/modulator/Upconverter/Carrier with Doppler/Intermediate Frequency ==
  Frame Clock : Inport
  Constant : Constant  Value=fc
  Gain4 : Gain  Gain=2*pi
  Product3 : Product
  IF Phase : Outport
  wires:
  Gain4/1 -> Product3/2
  Frame Clock/1 -> Product3/1
  Product3/1 -> IF Phase/1
  Constant/1 -> Gain4/1

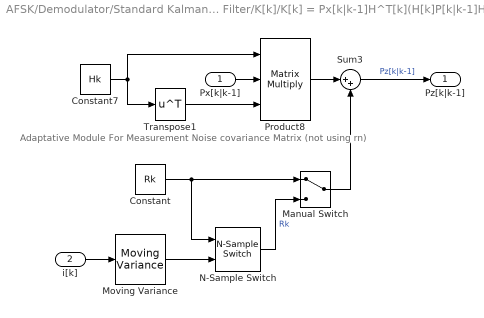
== system AFSK/Demodulator/Standard Kalman Filter/K[k]/K[k] = Px[k|k-1]H^T[k](H[k]P[k|k-1]H^T[k] + R[k])⁻¹ cf. (4.2.17) Brown/ Pz[k|k-1] = H[k] Px[k|k-1] H^T[k] + R[k] ==
  note: Adaptative Module
      | For Measurement Noise covariance Matrix (not using rn)
  Px[k|k-1] : Inport
  i[k] : Inport  Port=2
  Constant : Constant  Value=Rk
  Constant7 : Constant  Value=Hk  VectorParams1D=off  SampleTime=Tb
  Manual Switch : ManualSwitch
  Moving Variance : dspstat3/Moving Variance  Method=Sliding window  ForgettingFactorPort=off  SpecifyWindowLength=on  WindowLength=1000  OverlapLength=999  AllowArbitraryInputLength=off  ForgettingFactor=0.9  SimulateUsing=Interpreted execution
  N-Sample Switch : dspswit3/N-Sample Switch  N=3000  reset=off  TriggerType=Rising edge  Ts=Tb
  Product8 : Product  Inputs=3  Multiplication=Matrix(*)
  Sum3 : Sum  Inputs=|++
  Transpose1 : Math  Operator=transpose  SignedPower=on
  Pz[k|k-1] : Outport  VectorParamsAs1DForOutWhenUnconnected=off
  wires:
  Constant7/1 -> Transpose1/1, Product8/1
  Product8/1 -> Sum3/1
  Transpose1/1 -> Product8/3
  Sum3/1 -> Pz[k|k-1]/1  "Pz[k|k-1]"
  Px[k|k-1]/1 -> Product8/2
  i[k]/1 -> Moving Variance/1
  Moving Variance/1 -> N-Sample Switch/2
  N-Sample Switch/1 -> Manual Switch/2  "Rk"
  Constant/1 -> Manual Switch/1, N-Sample Switch/1
  Manual Switch/1 -> Sum3/2

== system AFSK/Demodulator/Standard Kalman Filter/K[k]/Px[k-1|k-1] Initialization/If Action Subsystem ==
  In1 : Inport
  Action Port : ActionPort
  Constant1 : Constant  Value=Px_0_0  VectorParams1D=off  SampleTime=Tb
  Constant3 : Constant  Value=zeros(M)  VectorParams1D=off  SampleTime=Tb
  Manual Switch : ManualSwitch  CurrentSetting=0
  N-Sample Switch1 : dspswit3/N-Sample Switch  N=26  reset=off  TriggerType=Rising edge  Ts=Tb
  Out1 : Outport
  wires:
  Manual Switch/1 -> N-Sample Switch1/1
  N-Sample Switch1/1 -> Out1/1
  In1/1 -> N-Sample Switch1/2
  Constant3/1 -> Manual Switch/1
  Constant1/1 -> Manual Switch/2

== system AFSK/Demodulator/Standard Kalman Filter/K[k]/Px[k-1|k-1] Initialization/If Action Subsystem1 ==
  In1 : Inport
  Action Port : ActionPort
  Out1 : Outport
  wires:
  In1/1 -> ?  "Px[k-1|k-1]"
  ? -> Out1/1

== system AFSK/modulator/Upconverter/Carrier with Doppler/Doppler Effect/Realistic Doppler ==
  Delay : Delay  DelayLength=1  InitialCondition=initial_estimates(1)
  From Workspace : FromWorkspace  VariableName=real_LOS_phase  SampleTime=Tb
  Linear Interpolation : MATLAB Function  TreatAsAtomicUnit=on
  Real LOS phase : Outport
  wires:
  Linear Interpolation/1(y) -> Real LOS phase/1  "Real LOS phase"
  Delay/1 -> Linear Interpolation/2(data_delayed)
  From Workspace/1 -> Linear Interpolation/1(data), Delay/1  "real LOS phase"

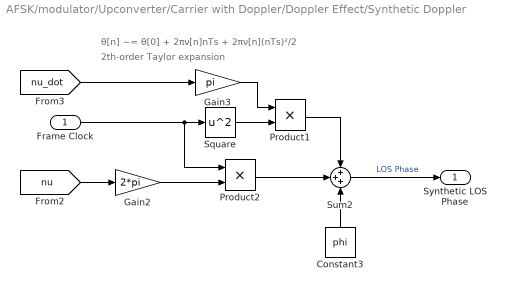
== system AFSK/modulator/Upconverter/Carrier with Doppler/Doppler Effect/Synthetic Doppler ==
  note: θ[n] ~= θ[0] + 2πν[n]nTs + 2πν[n](nTs)²/2
  note: 2th-order Taylor expansion
  Frame Clock : Inport
  Constant3 : Constant  Value=phi
  Gain2 : Gain  Gain=2*pi
  Gain3 : Gain  Gain=pi
  Product1 : Product
  Product2 : Product
  Square : Math  Operator=square
  Sum2 : Sum  Inputs=+++
  Synthetic LOS Phase : Outport
  wires:
  [nu] -> Gain2/1
  Gain2/1 -> Product2/2
  Frame Clock/1 -> Square/1, Product2/1
  Product1/1 -> Sum2/1
  [nu_dot] -> Gain3/1
  Square/1 -> Product1/2
  Constant3/1 -> Sum2/3
  Product2/1 -> Sum2/2
  Gain3/1 -> Product1/1
  Sum2/1 -> Synthetic LOS Phase/1  "LOS Phase"

== matlab function AFSK/timing delay/Linear Interpolation ==
  data: data input; data_delayed input; y output
function y = fcn(data, data_delayed)

y = interp1(0:1,[data_delayed,data],(0:400-1)/400,"linear").';

== matlab function AFSK/Demodulator/trace ==
  data: u input; y output
function y = fcn(u)

y = trace(u);

== matlab function AFSK/Demodulator/Standard Kalman Filter/MATLAB Function ==
  data: x00_init output; x00_matrix parameter; count data_store_memory; M parameter; init_LOS_delay parameter
function x00_init = fcn(x00_matrix,M, init_LOS_delay)
    global count
    if count <= 25 + init_LOS_delay + 1
        
        x00_init = x00_matrix(:,count);
    else
        x00_init = NaN(M,1);
    end
    count = count+1;
end

== matlab function AFSK/modulator/Doppler Effect/Realistic Doppler/Linear Interpolation ==
  data: data input; data_delayed input; y output
function y = fcn(data, data_delayed)

y = interp1(0:1,[data_delayed,data],(0:400-1)/400,"linear").';

== matlab function AFSK/Demodulator/Viterbi detector ==
  data: z1_s output; true_bit input; z1 input; z2 input; bit output size=1; metric_survivors data_store_memory; state data_store_memory; bits_window data_store_memory; depth data_store_memory; K parameter; z1_window data_store_memory; is_full_window data_store_memory; z2_window data_store_memory; terminal_phases parameter; z2_s output
function [z1_s, bit, z2_s] = viterbi_detector(true_bit, z1, z2, K, terminal_phases)
%% Initializing
global bits_window metric_survivors state depth z1_window z2_window is_full_window

%% resolving output
if is_full_window % bits_window is full
    % get the survivor metric, z1, and its respective transmitted bit
    [bit, z1_s, z2_s] = get_survivors(z1_window, z2_window, bits_window);
    
    % update the z1_window, z2_window, and bits_window
    [z1_window, z2_window, bits_window] = update_windows(z1_window, z2_window, bits_window);
else % bits_window is not full yet
    bit = NaN;
    z1_s = NaN;
    z2_s = complex(0);
end

%% Update the metrics
if isnan(true_bit)
    % perform the Viterbi algorithm. That is, save the metrics and detect the transmitted bit
    exp_terminal_phases = exp(-1j*terminal_phases);
    metrics = real(exp_terminal_phases .* z1);
    [bits_window, z1_window, z2_window, metric_survivors, state, depth, is_full_window] = viterbi_algorithm(metrics, bits_window, z1, z1_window, z2, z2_window, depth, K, metric_survivors, state);
else
    % use the true bit to decide z1 and z2. Hence, it doesn't save the metrics or detect the transmitted bit
    [bits_window, z1_window, z2_window, state, depth, is_full_window] = true_bit_algorithm(bits_window, true_bit, z1, z1_window, z2, z2_window, depth, K, state);
end

end

== matlab function AFSK/modulator/Upconverter/Carrier with Doppler/Doppler Effect/Realistic Doppler/Linear Interpolation ==
  data: data input; data_delayed input; y output
function y = fcn(data, data_delayed)

y = interp1(0:1,[data_delayed,data],(0:400-1)/400,"linear").';
